simulink model "LS_5_Replication"  (R2022a)
settings: Solver=ode45  StartTime=0.0  StopTime=SIM_DURATION  RelTol=1e-3
PreLoadFcn:
  | SAMPLE_TIME = 0.01;
  | X1_0               = 3;
  | X2_0               = -1;
undefined symbols (not defined in the file): ACI_actor_proj_eps, ACI_alpha, ACI_beta1, ACI_eta_a1, ACI_eta_a2, ACI_eta_c, ACI_gamma, ACI_Gamma_0, ACI_Gamma_vf, ACI_Gamma_wf, ACI_k, ACI_mu, ACI_Q, ACI_R, ACI_Wa_max_proj, DiscIntNeverNeededParam, W_Actor_0, W_Critic_0, X_0, X_dilde_0
settings Model: Creator=Z0150218  LastModifiedBy=Z0150218

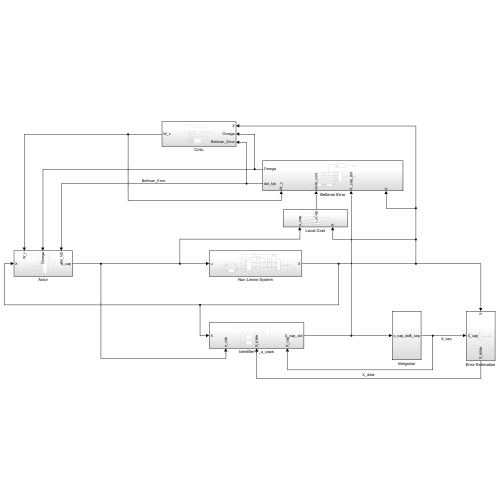
[thumbnail: Simulink's stored preview of the top-level diagram]
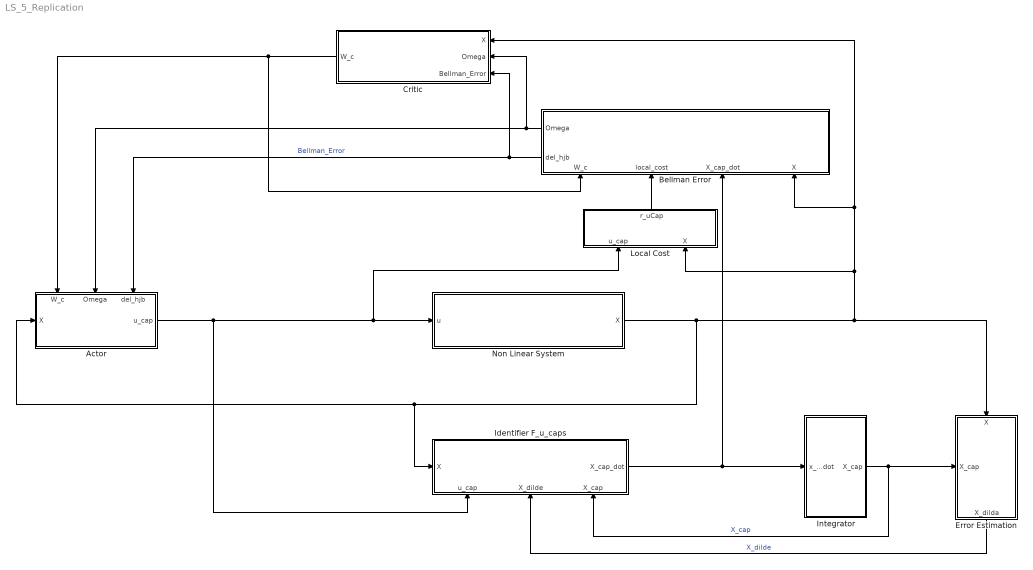
== system LS_5_Replication ==
  Actor : Subsystem
      settings: PortSchema="{\"entries\":[{\"content\":{\"sides\":[{\"content\":{\"connectorIds\":[\"In1\"]},\"type\":\"ConnectorPlacement.EquallySpacedRectSide\",\"uuid\":\"36bb19c7-ed28-4f81-a2b0-56b05d277fb3\"},{\"content\":{\"connectorIds\":[\"Out1\"],\"side\":\"RIGHT\"},\"type\":\"ConnectorPlacement.EquallySpacedRectSide\",\"uuid\":\"62e3b38d-27a4-411c-9c0c-4947886674bc\"},{\"content\":{\"connectorIds\":[\"In2\",\"In3\",\"In4\"],\"side\":\"TOP\"},\"type\":\"ConnectorPlacement.EquallySpacedRectSide\",\"uuid\":\"4750692c-c3eb-4933-9307-f150356a2a2d\"}]},\"type\":\"ConnectorPlacement.EquallySpacedConnector\",\"uuid\":\"9672208b-6d36-4217-80fb-cae3d46f9331\"}],\"packageUris\":[\"http://schema.mathworks.com/mf0/Connector/R2020b\"],\"version\":\"1.0\"}"
  Bellman Error : Subsystem
      settings: PortSchema="{\"entries\":[{\"content\":{\"sides\":[{\"content\":{\"connectorIds\":[]},\"type\":\"ConnectorPlacement.EquallySpacedRectSide\",\"uuid\":\"36bb19c7-ed28-4f81-a2b0-56b05d277fb3\"},{\"content\":{\"connectorIds\":[\"Out1\",\"Out2\"],\"side\":\"RIGHT\"},\"type\":\"ConnectorPlacement.EquallySpacedRectSide\",\"uuid\":\"62e3b38d-27a4-411c-9c0c-4947886674bc\"},{\"content\":{\"connectorIds\":[],\"side\":\"TOP\"},\"type\":\"ConnectorPlacement.EquallySpacedRectSide\",\"uuid\":\"4750692c-c3eb-4933-9307-f150356a2a2d\"},{\"content\":{\"connectorIds\":[\"In1\",\"In2\",\"In3\",\"In4\"],\"side\":\"BOTTOM\"},\"type\":\"ConnectorPlacement.EquallySpacedRectSide\",\"uuid\":\"b0657caa-1455-4a9e-81b4-6cca98e3a9da\"}]},\"type\":\"ConnectorPlacement.EquallySpacedConnector\",\"uuid\":\"9672208b-6d36-4217-80fb-cae3d46f9331\"}],\"packageUris\":[\"http://schema.mathworks.com/mf0/Connector/R2020b\"],\"version\":\"1.0\"}"
  Critic : Subsystem
  Error Estimation : Subsystem
      settings: PortSchema="{\"entries\":[{\"content\":{\"sides\":[{\"content\":{\"connectorIds\":[\"In1\"]},\"type\":\"ConnectorPlacement.EquallySpacedRectSide\",\"uuid\":\"e6cf2d84-7a10-4a43-bedd-b04786a9576e\"},{\"content\":{\"connectorIds\":[],\"side\":\"RIGHT\"},\"type\":\"ConnectorPlacement.EquallySpacedRectSide\",\"uuid\":\"10774151-562d-4d84-8145-e832c7227519\"},{\"content\":{\"connectorIds\":[\"In2\"],\"side\":\"TOP\"},\"type\":\"ConnectorPlacement.EquallySpacedRectSide\",\"uuid\":\"9da06394-e71b-407b-8c05-fa01b9a02c64\"},{\"content\":{\"connectorIds\":[\"Out1\"],\"side\":\"BOTTOM\"},\"type\":\"ConnectorPlacement.EquallySpacedRectSide\",\"uuid\":\"810c4029-0c70-4755-acf7-2aa0685db048\"}]},\"type\":\"ConnectorPlacement.EquallySpacedConnector\",\"uuid\":\"62376291-d5b3-4405-a096-61004334c23a\"}],\"packageUris\":[\"http://schema.mathworks.com/mf0/Connector/R2020b\"],\"version\":\"1.0\"}"
  Identifier F_u_caps : Subsystem
      settings: PortSchema="{\"entries\":[{\"content\":{\"sides\":[{\"content\":{\"connectorIds\":[\"In1\"]},\"type\":\"ConnectorPlacement.EquallySpacedRectSide\",\"uuid\":\"36bb19c7-ed28-4f81-a2b0-56b05d277fb3\"},{\"content\":{\"connectorIds\":[\"Out1\"],\"side\":\"RIGHT\"},\"type\":\"ConnectorPlacement.EquallySpacedRectSide\",\"uuid\":\"62e3b38d-27a4-411c-9c0c-4947886674bc\"},{\"content\":{\"connectorIds\":[],\"side\":\"TOP\"},\"type\":\"ConnectorPlacement.EquallySpacedRectSide\",\"uuid\":\"4750692c-c3eb-4933-9307-f150356a2a2d\"},{\"content\":{\"connectorIds\":[\"In2\",\"In3\",\"In4\"],\"side\":\"BOTTOM\"},\"type\":\"ConnectorPlacement.EquallySpacedRectSide\",\"uuid\":\"846bc86a-ab95-449a-8b91-40ba4137f590\"}]},\"type\":\"ConnectorPlacement.EquallySpacedConnector\",\"uuid\":\"9672208b-6d36-4217-80fb-cae3d46f9331\"}],\"packageUris\":[\"http://schema.mathworks.com/mf0/Connector/R2020b\"],\"version\":\"1.0\"}"
  Integrator : Subsystem
  Local Cost : Subsystem
      settings: PortSchema="{\"entries\":[{\"content\":{\"sides\":[{\"content\":{\"connectorIds\":[]},\"type\":\"ConnectorPlacement.EquallySpacedRectSide\",\"uuid\":\"36bb19c7-ed28-4f81-a2b0-56b05d277fb3\"},{\"content\":{\"connectorIds\":[],\"side\":\"RIGHT\"},\"type\":\"ConnectorPlacement.EquallySpacedRectSide\",\"uuid\":\"62e3b38d-27a4-411c-9c0c-4947886674bc\"},{\"content\":{\"connectorIds\":[\"Out1\"],\"side\":\"TOP\"},\"type\":\"ConnectorPlacement.EquallySpacedRectSide\",\"uuid\":\"4750692c-c3eb-4933-9307-f150356a2a2d\"},{\"content\":{\"connectorIds\":[\"In1\",\"In2\"],\"side\":\"BOTTOM\"},\"type\":\"ConnectorPlacement.EquallySpacedRectSide\",\"uuid\":\"45987bb4-5db5-4673-a5e8-75a3f7947a65\"}]},\"type\":\"ConnectorPlacement.EquallySpacedConnector\",\"uuid\":\"9672208b-6d36-4217-80fb-cae3d46f9331\"}],\"packageUris\":[\"http://schema.mathworks.com/mf0/Connector/R2020b\"],\"version\":\"1.0\"}"
  Non Linear System : Subsystem
  wires:
  Actor/1(u_cap) -> Non Linear System/1(u), Local Cost/1(u_cap), Identifier F_u_caps/2(u_cap)
  Identifier F_u_caps/1(X_cap_dot) -> Integrator/1(x_cap_dot), Bellman Error/2(X_cap_dot)
  Integrator/1(X_cap) -> Identifier F_u_caps/4(X_cap), Error Estimation/1(X_cap)  "X_cap"
  Non Linear System/1(X) -> Identifier F_u_caps/1(X), Actor/1(X), Bellman Error/1(X), Critic/1(X), Local Cost/2(X), Error Estimation/2(X)
  Critic/1(W_c) -> Actor/2(W_c), Bellman Error/4(W_c)
  Local Cost/1(r_uCap) -> Bellman Error/3(local_cost)
  Error Estimation/1(X_dilda) -> Identifier F_u_caps/3(X_dilde)  "X_dilde"
  Bellman Error/2(del_hjb) -> Critic/3(Bellman_Error), Actor/4(del_hjb)  "Bellman_Error"
  Bellman Error/1(Omega) -> Actor/3(Omega), Critic/2(Omega)

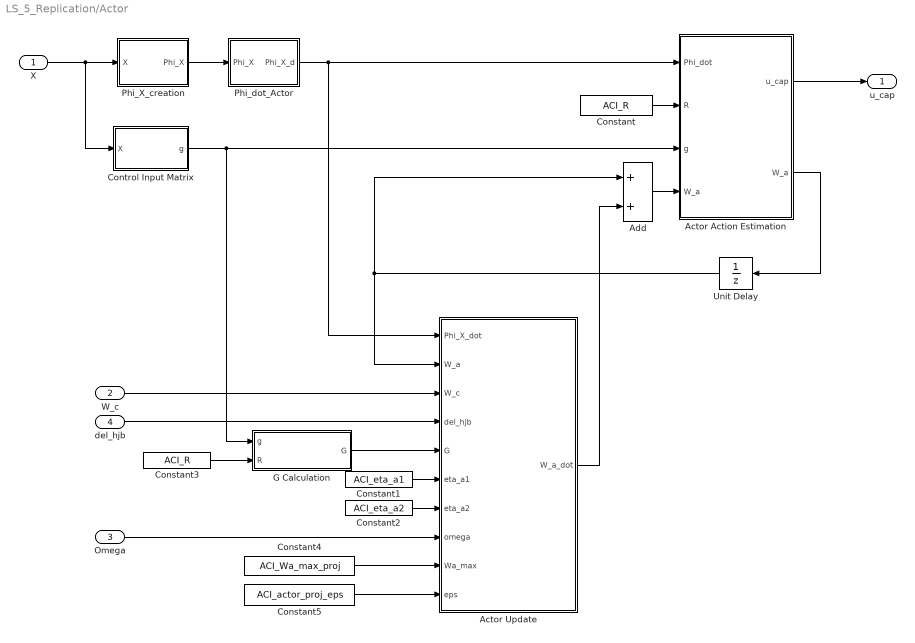
== system LS_5_Replication/Actor ==
  X : Inport
  W_c : Inport  Port=2
  Omega : Inport  Port=3
  del_hjb : Inport  Port=4
  Actor Action Estimation : MATLAB Function  TreatAsAtomicUnit=on
  Actor Update : MATLAB Function  TreatAsAtomicUnit=on
  Add : Sum
  Constant : Constant  Value=ACI_R
  Constant1 : Constant  Value=ACI_eta_a1
  Constant2 : Constant  Value=ACI_eta_a2
  Constant3 : Constant  Value=ACI_R
  Constant4 : Constant  Value=ACI_Wa_max_proj
  Constant5 : Constant  Value=ACI_actor_proj_eps
  Control Input Matrix : MATLAB Function  TreatAsAtomicUnit=on
  G Calculation : MATLAB Function  TreatAsAtomicUnit=on
  Phi_X_creation : MATLAB Function  TreatAsAtomicUnit=on
  Phi_dot_Actor : Subsystem
  Unit Delay : UnitDelay  InitialCondition=W_Actor_0  SampleTime=SAMPLE_TIME  HasFrameUpgradeWarning=on
  u_cap : Outport
  wires:
  Actor Action Estimation/2(W_a) -> Unit Delay/1
  Constant/1 -> Actor Action Estimation/2(R)
  Control Input Matrix/1(g) -> G Calculation/1(g), Actor Action Estimation/3(g)
  del_hjb/1 -> Actor Update/4(del_hjb)
  W_c/1 -> Actor Update/3(W_c)
  Unit Delay/1 -> Add/1, Actor Update/2(W_a)
  Actor Update/1(W_a_dot) -> Add/2
  Add/1 -> Actor Action Estimation/4("W_a ")
  X/1 -> Control Input Matrix/1(X), Phi_X_creation/1(X)
  Phi_X_creation/1(Phi_X) -> Phi_dot_Actor/1(Phi_X)
  Constant1/1 -> Actor Update/6(eta_a1)
  Constant2/1 -> Actor Update/7(eta_a2)
  Omega/1 -> Actor Update/8(omega)
  G Calculation/1(G) -> Actor Update/5(G)
  Constant3/1 -> G Calculation/2(R)
  Phi_dot_Actor/1(Phi_X_d) -> Actor Update/1(Phi_X_dot), Actor Action Estimation/1(Phi_dot)
  Actor Action Estimation/1(u_cap) -> u_cap/1
  Constant4/1 -> Actor Update/9(Wa_max)
  Constant5/1 -> Actor Update/10(eps)

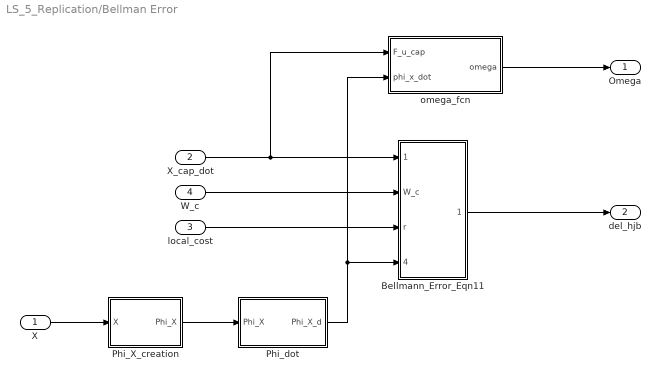
== system LS_5_Replication/Bellman Error ==
  X : Inport
  X_cap_dot : Inport  Port=2
  local_cost : Inport  Port=3
  W_c : Inport  Port=4
  Bellmann_Error_Eqn11 : MATLAB Function  TreatAsAtomicUnit=on
  Phi_X_creation : MATLAB Function  TreatAsAtomicUnit=on
  Phi_dot : Subsystem
  omega_fcn : MATLAB Function  TreatAsAtomicUnit=on
  Omega : Outport
  del_hjb : Outport  Port=2
  wires:
  X/1 -> Phi_X_creation/1(X)
  Phi_X_creation/1(Phi_X) -> Phi_dot/1(Phi_X)
  local_cost/1 -> Bellmann_Error_Eqn11/3(r)
  W_c/1 -> Bellmann_Error_Eqn11/2(W_c)
  X_cap_dot/1 -> Bellmann_Error_Eqn11/1(F_u_cap), omega_fcn/1(F_u_cap)
  Bellmann_Error_Eqn11/1(del_hjb) -> del_hjb/1
  Phi_dot/1(Phi_X_d) -> Bellmann_Error_Eqn11/4(phi_x_d), omega_fcn/2(phi_x_dot)
  omega_fcn/1(omega) -> Omega/1

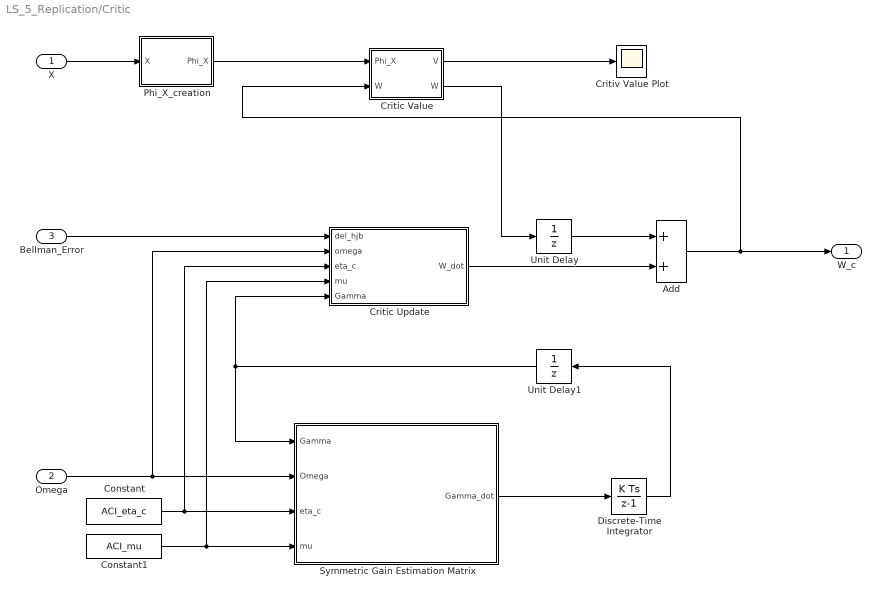
== system LS_5_Replication/Critic ==
  X : Inport
  Omega : Inport  Port=2
  Bellman_Error : Inport  Port=3
  Add : Sum
  Constant : Constant  Value=ACI_eta_c
  Constant1 : Constant  Value=ACI_mu
  Critic Update : MATLAB Function  TreatAsAtomicUnit=on
  Critic Value : MATLAB Function  TreatAsAtomicUnit=on
  Critiv Value Plot : Scope
  Discrete-Time Integrator : DiscreteIntegrator  InitialCondition=ACI_Gamma_0  SampleTime=-1  ICPrevOutput=DiscIntNeverNeededParam  ICPrevScaledInput=DiscIntNeverNeededParam
  Phi_X_creation : MATLAB Function  TreatAsAtomicUnit=on
  Symmetric Gain Estimation Matrix : MATLAB Function  TreatAsAtomicUnit=on
  Unit Delay : UnitDelay  InitialCondition=W_Critic_0  SampleTime=SAMPLE_TIME  HasFrameUpgradeWarning=on
  Unit Delay1 : UnitDelay  SampleTime=-1  HasFrameUpgradeWarning=on
  W_c : Outport
  wires:
  Critic Value/1(V) -> Critiv Value Plot/1
  Add/1 -> Critic Value/2("W "), W_c/1
  X/1 -> Phi_X_creation/1(X)
  Critic Value/2(W) -> Unit Delay/1
  Critic Update/1(W_dot) -> Add/2
  Bellman_Error/1 -> Critic Update/1(del_hjb)
  Unit Delay/1 -> Add/1
  Phi_X_creation/1(Phi_X) -> Critic Value/1(Phi_X)
  Symmetric Gain Estimation Matrix/1(Gamma_dot) -> Discrete-Time Integrator/1
  Discrete-Time Integrator/1 -> Unit Delay1/1
  Omega/1 -> Critic Update/2(omega), Symmetric Gain Estimation Matrix/2(Omega)
  Constant/1 -> Critic Update/3(eta_c), Symmetric Gain Estimation Matrix/3(eta_c)
  Constant1/1 -> Critic Update/4(mu), Symmetric Gain Estimation Matrix/4(mu)
  Unit Delay1/1 -> Critic Update/5(Gamma), Symmetric Gain Estimation Matrix/1(Gamma)

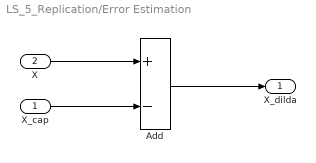
== system LS_5_Replication/Error Estimation ==
  X_cap : Inport
  X : Inport  Port=2
  Add : Sum  Inputs=+-
  X_dilda : Outport
  wires:
  Add/1 -> X_dilda/1
  X/1 -> Add/1
  X_cap/1 -> Add/2

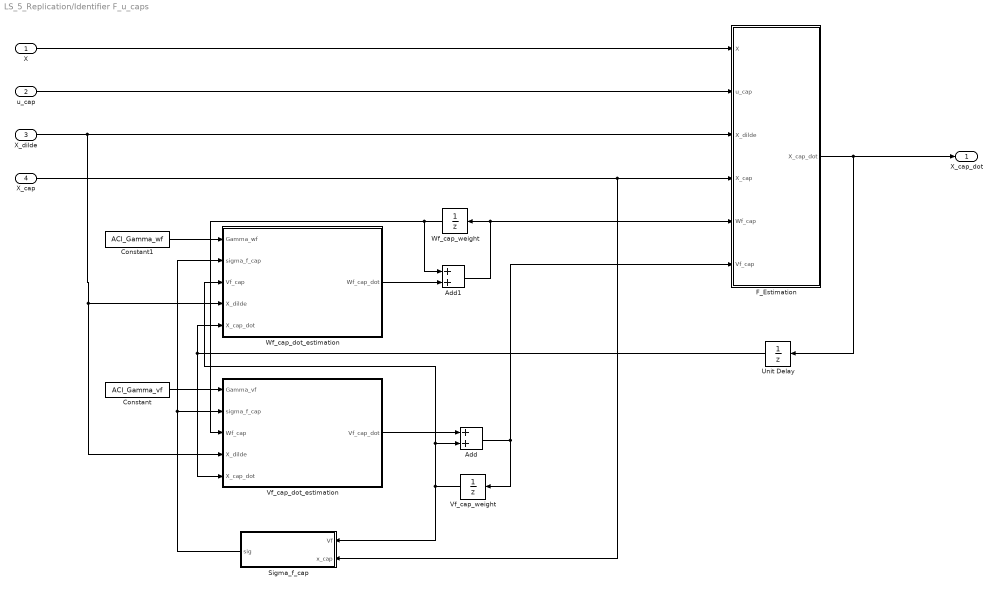
== system LS_5_Replication/Identifier F_u_caps ==
  X : Inport
  u_cap : Inport  Port=2
  X_dilde : Inport  Port=3
  X_cap : Inport  Port=4
  Add : Sum
  Add1 : Sum
  Constant : Constant  Value=ACI_Gamma_vf
  Constant1 : Constant  Value=ACI_Gamma_wf
  F_Estimation : Subsystem
  Sigma_f_cap : MATLAB Function  TreatAsAtomicUnit=on
  Unit Delay : UnitDelay  SampleTime=-1  HasFrameUpgradeWarning=on
  Vf_cap_dot_estimation : MATLAB Function  TreatAsAtomicUnit=on
  Vf_cap_weight : UnitDelay  SampleTime=-1  HasFrameUpgradeWarning=on
  Wf_cap_dot_estimation : MATLAB Function  TreatAsAtomicUnit=on
  Wf_cap_weight : UnitDelay  SampleTime=-1  HasFrameUpgradeWarning=on
  X_cap_dot : Outport
  wires:
  u_cap/1 -> F_Estimation/2(u_cap)
  X_dilde/1 -> Vf_cap_dot_estimation/4(X_dilde), Wf_cap_dot_estimation/4(X_dilde), F_Estimation/3(X_dilde)
  X_cap/1 -> Sigma_f_cap/2(x_cap), F_Estimation/4(X_cap)
  Wf_cap_dot_estimation/1(Wf_cap_dot) -> Add1/2
  Constant1/1 -> Wf_cap_dot_estimation/1(Gamma_wf)
  Vf_cap_dot_estimation/1(Vf_cap_dot) -> Add/1
  Constant/1 -> Vf_cap_dot_estimation/1(Gamma_vf)
  Add/1 -> F_Estimation/6(Vf_cap), Vf_cap_weight/1
  Add1/1 -> Wf_cap_weight/1, F_Estimation/5(Wf_cap)
  Vf_cap_weight/1 -> Wf_cap_dot_estimation/3(Vf_cap), Add/2, Sigma_f_cap/1(Vf)
  Wf_cap_weight/1 -> Add1/1, Vf_cap_dot_estimation/3(Wf_cap)
  X/1 -> F_Estimation/1(X)
  Sigma_f_cap/1(sig) -> Vf_cap_dot_estimation/2(sigma_f_cap), Wf_cap_dot_estimation/2(sigma_f_cap)
  F_Estimation/1(X_cap_dot) -> X_cap_dot/1, Unit Delay/1
  Unit Delay/1 -> Vf_cap_dot_estimation/5(X_cap_dot), Wf_cap_dot_estimation/5(X_cap_dot)

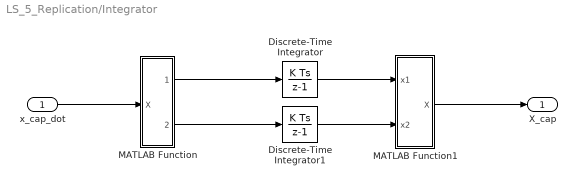
== system LS_5_Replication/Integrator ==
  x_cap_dot : Inport
  Discrete-Time Integrator : DiscreteIntegrator  SampleTime=SAMPLE_TIME  ICPrevOutput=DiscIntNeverNeededParam  ICPrevScaledInput=DiscIntNeverNeededParam
  Discrete-Time Integrator1 : DiscreteIntegrator  SampleTime=SAMPLE_TIME  ICPrevOutput=DiscIntNeverNeededParam  ICPrevScaledInput=DiscIntNeverNeededParam
  MATLAB Function : MATLAB Function  TreatAsAtomicUnit=on
  MATLAB Function1 : MATLAB Function  TreatAsAtomicUnit=on
  X_cap : Outport
  wires:
  x_cap_dot/1 -> MATLAB Function/1(X)
  MATLAB Function/1(x1) -> Discrete-Time Integrator/1
  MATLAB Function/2(x2) -> Discrete-Time Integrator1/1
  Discrete-Time Integrator/1 -> MATLAB Function1/1(x1)
  Discrete-Time Integrator1/1 -> MATLAB Function1/2(x2)
  MATLAB Function1/1(X) -> X_cap/1

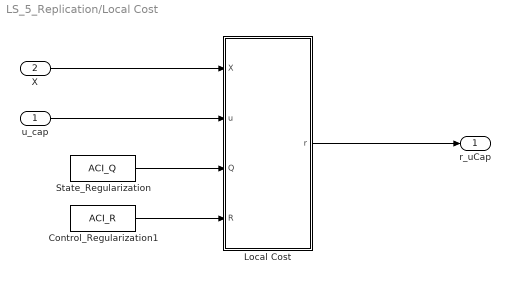
== system LS_5_Replication/Local Cost ==
  u_cap : Inport
  X : Inport  Port=2
  Control_Regularization1 : Constant  Value=ACI_R
  Local Cost : MATLAB Function  TreatAsAtomicUnit=on
  State_Regularization : Constant  Value=ACI_Q
  r_uCap : Outport
  wires:
  u_cap/1 -> Local Cost/2(u)
  X/1 -> Local Cost/1(X)
  State_Regularization/1 -> Local Cost/3(Q)
  Control_Regularization1/1 -> Local Cost/4(R)
  Local Cost/1(r) -> r_uCap/1

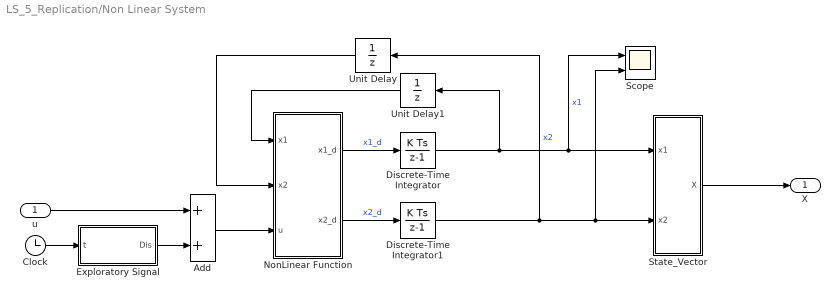
== system LS_5_Replication/Non Linear System ==
  u : Inport
  Add : Sum
  Clock : Clock
  Discrete-Time Integrator : DiscreteIntegrator  InitialCondition=X_0(1)  SampleTime=SAMPLE_TIME  ICPrevOutput=DiscIntNeverNeededParam  ICPrevScaledInput=DiscIntNeverNeededParam
  Discrete-Time Integrator1 : DiscreteIntegrator  InitialCondition=X_0(2)  SampleTime=SAMPLE_TIME  ICPrevOutput=DiscIntNeverNeededParam  ICPrevScaledInput=DiscIntNeverNeededParam
  Exploratory Signal : MATLAB Function  TreatAsAtomicUnit=on
  NonLinear Function : MATLAB Function  TreatAsAtomicUnit=on
  Scope : Scope  NumInputPorts=2
  State_Vector : MATLAB Function  TreatAsAtomicUnit=on
  Unit Delay : UnitDelay  SampleTime=-1  HasFrameUpgradeWarning=on
  Unit Delay1 : UnitDelay  SampleTime=-1  HasFrameUpgradeWarning=on
  X : Outport
  wires:
  Discrete-Time Integrator1/1 -> Unit Delay/1, Scope/2, State_Vector/2(x2)  "x2"
  NonLinear Function/2(x2_d) -> Discrete-Time Integrator1/1  "x2_d"
  NonLinear Function/1(x1_d) -> Discrete-Time Integrator/1  "x1_d"
  Discrete-Time Integrator/1 -> State_Vector/1(x1), Scope/1, Unit Delay1/1  "x1"
  State_Vector/1(X) -> X/1
  u/1 -> Add/1
  Unit Delay1/1 -> NonLinear Function/1(x1)
  Unit Delay/1 -> NonLinear Function/2(x2)
  Clock/1 -> Exploratory Signal/1(t)
  Exploratory Signal/1(Dis) -> Add/2
  Add/1 -> NonLinear Function/3(u)

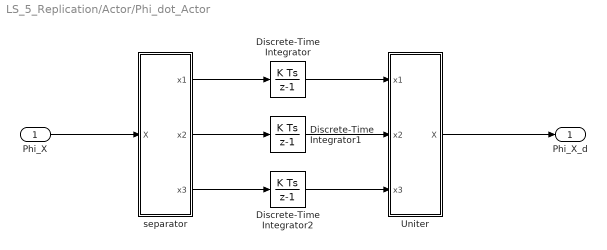
== system LS_5_Replication/Actor/Phi_dot_Actor ==
  Phi_X : Inport
  Discrete-Time Integrator : DiscreteIntegrator  SampleTime=-1  ICPrevOutput=DiscIntNeverNeededParam  ICPrevScaledInput=DiscIntNeverNeededParam
  Discrete-Time Integrator1 : DiscreteIntegrator  SampleTime=-1  ICPrevOutput=DiscIntNeverNeededParam  ICPrevScaledInput=DiscIntNeverNeededParam
  Discrete-Time Integrator2 : DiscreteIntegrator  SampleTime=-1  ICPrevOutput=DiscIntNeverNeededParam  ICPrevScaledInput=DiscIntNeverNeededParam
  Uniter : MATLAB Function  TreatAsAtomicUnit=on
  separator : MATLAB Function  TreatAsAtomicUnit=on
  Phi_X_d : Outport
  wires:
  Phi_X/1 -> separator/1(X)
  separator/1(x1) -> Discrete-Time Integrator/1
  separator/3(x3) -> Discrete-Time Integrator2/1
  separator/2(x2) -> Discrete-Time Integrator1/1
  Discrete-Time Integrator/1 -> Uniter/1(x1)
  Discrete-Time Integrator1/1 -> Uniter/2(x2)
  Discrete-Time Integrator2/1 -> Uniter/3(x3)
  Uniter/1(X) -> Phi_X_d/1

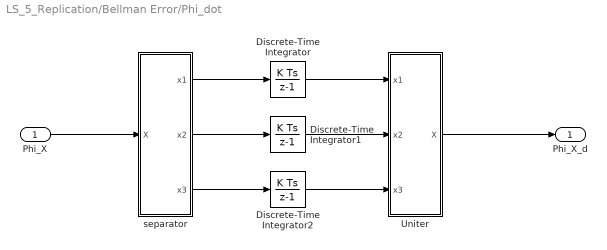
== system LS_5_Replication/Bellman Error/Phi_dot ==
  Phi_X : Inport
  Discrete-Time Integrator : DiscreteIntegrator  SampleTime=-1  ICPrevOutput=DiscIntNeverNeededParam  ICPrevScaledInput=DiscIntNeverNeededParam
  Discrete-Time Integrator1 : DiscreteIntegrator  SampleTime=-1  ICPrevOutput=DiscIntNeverNeededParam  ICPrevScaledInput=DiscIntNeverNeededParam
  Discrete-Time Integrator2 : DiscreteIntegrator  SampleTime=-1  ICPrevOutput=DiscIntNeverNeededParam  ICPrevScaledInput=DiscIntNeverNeededParam
  Uniter : MATLAB Function  TreatAsAtomicUnit=on
  separator : MATLAB Function  TreatAsAtomicUnit=on
  Phi_X_d : Outport
  wires:
  Phi_X/1 -> separator/1(X)
  separator/1(x1) -> Discrete-Time Integrator/1
  separator/3(x3) -> Discrete-Time Integrator2/1
  separator/2(x2) -> Discrete-Time Integrator1/1
  Discrete-Time Integrator/1 -> Uniter/1(x1)
  Discrete-Time Integrator1/1 -> Uniter/2(x2)
  Discrete-Time Integrator2/1 -> Uniter/3(x3)
  Uniter/1(X) -> Phi_X_d/1

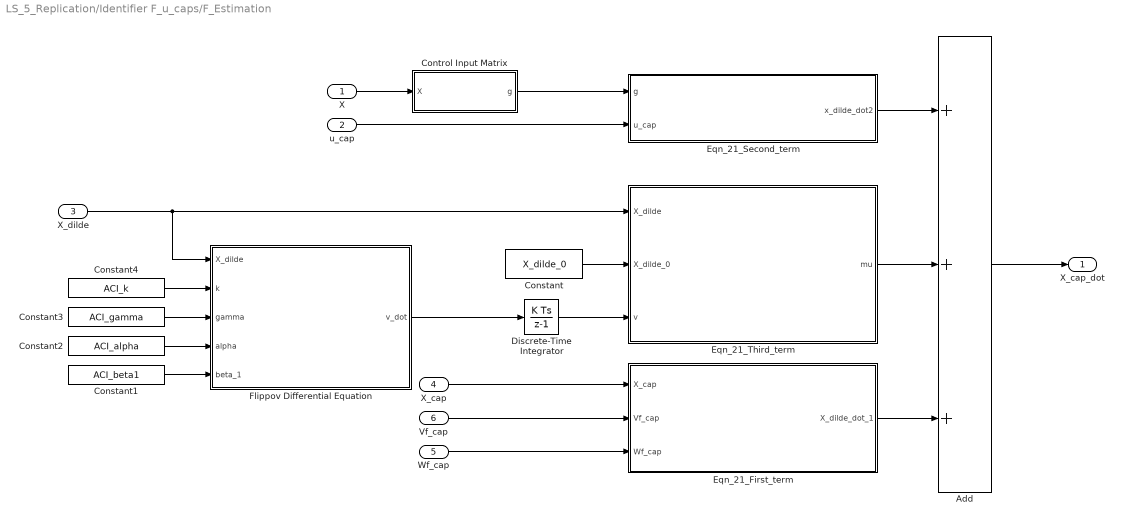
== system LS_5_Replication/Identifier F_u_caps/F_Estimation ==
  X : Inport
  u_cap : Inport  Port=2
  X_dilde : Inport  Port=3
  X_cap : Inport  Port=4
  Wf_cap : Inport  Port=5
  Vf_cap : Inport  Port=6
  Add : Sum  Inputs=+++
  Constant : Constant  Value=X_dilde_0
  Constant1 : Constant  Value=ACI_beta1
  Constant2 : Constant  Value=ACI_alpha
  Constant3 : Constant  Value=ACI_gamma
  Constant4 : Constant  Value=ACI_k
  Control Input Matrix : MATLAB Function  TreatAsAtomicUnit=on
  Discrete-Time Integrator : DiscreteIntegrator  SampleTime=SAMPLE_TIME  ICPrevOutput=DiscIntNeverNeededParam  ICPrevScaledInput=DiscIntNeverNeededParam
  Eqn_21_First_term : MATLAB Function  TreatAsAtomicUnit=on
  Eqn_21_Second_term : MATLAB Function  TreatAsAtomicUnit=on
  Eqn_21_Third_term : MATLAB Function  TreatAsAtomicUnit=on
  Flippov Differential Equation : MATLAB Function  TreatAsAtomicUnit=on
  X_cap_dot : Outport
  wires:
  Vf_cap/1 -> Eqn_21_First_term/2(Vf_cap)
  X_dilde/1 -> Flippov Differential Equation/1(X_dilde), Eqn_21_Third_term/1(X_dilde)
  Discrete-Time Integrator/1 -> Eqn_21_Third_term/3(v)
  Eqn_21_Second_term/1(x_dilde_dot2) -> Add/1
  X_cap/1 -> Eqn_21_First_term/1(X_cap)
  Constant/1 -> Eqn_21_Third_term/2(X_dilde_0)
  Eqn_21_First_term/1(X_dilde_dot_1) -> Add/3
  Flippov Differential Equation/1(v_dot) -> Discrete-Time Integrator/1
  Eqn_21_Third_term/1(mu) -> Add/2
  Add/1 -> X_cap_dot/1
  Wf_cap/1 -> Eqn_21_First_term/3(Wf_cap)
  u_cap/1 -> Eqn_21_Second_term/2(u_cap)
  X/1 -> Control Input Matrix/1(X)
  Control Input Matrix/1(g) -> Eqn_21_Second_term/1(g)
  Constant1/1 -> Flippov Differential Equation/5(beta_1)
  Constant2/1 -> Flippov Differential Equation/4(alpha)
  Constant3/1 -> Flippov Differential Equation/3(gamma)
  Constant4/1 -> Flippov Differential Equation/2(k)

== matlab function LS_5_Replication/Identifier F_u_caps/F_Estimation/Flippov Differential Equation ==
  data: X_dilde input; v_dot output; k input; gamma input; alpha input; beta_1 input
function v_dot = Flippov_GS(X_dilde, k, gamma, alpha, beta_1)

v_dot_1                = ((k*alpha) + gamma) * X_dilde;
v_dot_2                = beta_1 * sign(X_dilde);
v_dot                  = v_dot_1 + v_dot_2;

== matlab function LS_5_Replication/Identifier F_u_caps/F_Estimation/Eqn_21_First_term ==
  data: X_cap input; X_dilde_dot_1 output; Vf_cap input; Wf_cap input
function X_dilde_dot_1  = DNN(X_cap, Vf_cap, Wf_cap)

term1            = Vf_cap'*X_cap;
sigma_f_cap      = fcn_ACI_DNN_Activation(term1);
X_dilde_dot_1    = Wf_cap'*sigma_f_cap;
end

== matlab function LS_5_Replication/Identifier F_u_caps/Wf_cap_dot_estimation ==
  data: Gamma_wf input; Wf_cap_dot output; sigma_f_cap input; Vf_cap input; X_dilde input; X_cap_dot input
function Wf_cap_dot = Wf_cap_d_Est(Gamma_wf, sigma_f_cap,Vf_cap,X_dilde,X_cap_dot)


Proj              = 1;
Wf_cap_dot_t      = Proj*Gamma_wf*sigma_f_cap'*Vf_cap'*X_cap_dot*X_dilde';
Wf_cap_dot        = Wf_cap_dot_t;
end

== matlab function LS_5_Replication/Identifier F_u_caps/Vf_cap_dot_estimation ==
  data: Gamma_vf input; Vf_cap_dot output; sigma_f_cap input; Wf_cap input; X_dilde input; X_cap_dot input
function Vf_cap_dot = Vf_cap_d_Est(Gamma_vf, sigma_f_cap,Wf_cap,X_dilde,X_cap_dot)


Proj              = 1;
Vf_cap_dot        = Proj*Gamma_vf*X_cap_dot*X_dilde'*Wf_cap'*sigma_f_cap';

end

== matlab function LS_5_Replication/Local Cost/Local Cost ==
  data: X input; u input; r output; Q input; R input
function r = Local_Cost(X,u,Q,R)

elem1     = u'*R*u;
elem2     = X'*Q*X;
r         = elem1 + elem2;
end

== matlab function LS_5_Replication/Bellman Error/Bellmann_Error_Eqn11 ==
  data: F_u_cap input; W_c input; del_hjb output; r input; phi_x_d input
function del_hjb = hjb(F_u_cap,W_c,r,phi_x_d)

omega   = phi_x_d * F_u_cap; 
del_hjb = (W_c'*omega) + r;
end

== matlab function LS_5_Replication/Critic/Critic Value ==
  data: Phi_X input; W input; V output; W output
function [V,W] = Critic(Phi_X,W)


V     = W'*Phi_X;  % Equation 10
end

== matlab function LS_5_Replication/Integrator/MATLAB Function ==
  data: X input; x1 output; x2 output
function [x1,x2] = fcn(X)

x1 = X(1);
x2 = X(2);
end

== matlab function LS_5_Replication/Integrator/MATLAB Function1 ==
  data: x1 input; X output; x2 input
function X = fcn(x1,x2)

X = [x1; x2];

== matlab function LS_5_Replication/Bellman Error/Phi_X_creation ==
  data: X input; Phi_X output
function Phi_X = fcn_ACI_Phi(X)
px1   = X(1)^2;
px2   = X(1)*X(2);
px3   = X(2)^2;
Phi_X = [px1; px2; px3];

end

== matlab function LS_5_Replication/Bellman Error/Phi_dot/separator ==
  data: X input; x1 output; x2 output; x3 output
function [x1,x2,x3] = fcn(X)

x1 = X(1);
x2 = X(2);
x3 = X(3);
end

== matlab function LS_5_Replication/Bellman Error/Phi_dot/Uniter ==
  data: x1 input; X output; x2 input; x3 input
function X  = fcn(x1,x2,x3)

X = [x1 x1; x2 x2; x3 x3];
end

== matlab function LS_5_Replication/Non Linear System/State_Vector ==
  data: x1 input; X output; x2 input
function X = fcn(x1,x2)

X = [x1; x2];

end

== matlab function LS_5_Replication/Critic/Phi_X_creation ==
  data: X input; Phi_X output
function Phi_X = fcn_ACI_Phi(X)
px1   = X(1)^2;
px2   = X(1)*X(2);
px3   = X(2)^2;
Phi_X = [px1; px2; px3];

end

== matlab function LS_5_Replication/Actor/Phi_X_creation ==
  data: X input; Phi_X output
function Phi_X = fcn_ACI_Phi(X)
px1   = X(1)^2;
px2   = X(1)*X(2);
px3   = X(2)^2;
Phi_X = [px1; px2; px3];

end

== matlab function LS_5_Replication/Critic/Symmetric Gain Estimation Matrix ==
  data: Gamma input; Gamma_dot output; Omega input; eta_c input; mu input
function Gamma_dot = Gain_Matrix(Gamma,Omega,eta_c,mu)

num         = Omega*Omega';
den         = 1 + (mu*Omega'*Gamma*Omega);

temp        = num/den;

Gamma_dot   = -eta_c*Gamma*temp*Gamma;


end

== matlab function LS_5_Replication/Bellman Error/omega_fcn ==
  data: F_u_cap input; phi_x_dot input; omega output
function omega = fcn(F_u_cap, phi_x_dot)

omega = phi_x_dot*F_u_cap;
end

== matlab function LS_5_Replication/Actor/Phi_dot_Actor/Uniter ==
  data: x1 input; X output; x2 input; x3 input
function X  = fcn(x1,x2,x3)

X = [x1 x1; x2 x2; x3 x3];
end

== matlab function LS_5_Replication/Non Linear System/NonLinear Function ==
  data: x1 input; x2 input; u input; x1_d output; x2_d output
function [x1_d, x2_d] = Non_Linear(x1,x2,u)

x1_d = -x1 + x2;
x2_d = (-0.5*x1) - (0.5*x2*(1 - (cos(2*x1)+2)^2)) + (cos(2*x1)+2)*u;
end

== matlab function LS_5_Replication/Actor/Phi_dot_Actor/separator ==
  data: X input; x1 output; x2 output; x3 output
function [x1,x2,x3] = fcn(X)

x1 = X(1);
x2 = X(2);
x3 = X(3);
end

== matlab function LS_5_Replication/Actor/G Calculation ==
  data: g input; G output; R input
function G = G_symmetric(g,R)

term1 = R\g;
G     = term1*g';
end

== matlab function LS_5_Replication/Non Linear System/Exploratory Signal ==
  data: t input; Dis output
function Dis = PE(t)

if t <= 3
    tm1 = cos(t)*(sin(t)^2);
    tm2 = cos(0.1*t)*(sin(2*t)^2);
    tm3 = cos(0.5*t)*(sin(-1.2*t)^2);
    tm4 = sin(t)^5;
    Dis = tm1 + tm2 +tm3 + tm4;
else
    Dis = 0;
end

== matlab function LS_5_Replication/Identifier F_u_caps/Sigma_f_cap ==
  data: Vf input; sig output; x_cap input
function sig = Sigma_f_cap(Vf,x_cap)

sig = fcn_ACI_DNN_Activation(Vf'*x_cap);
end

== matlab function LS_5_Replication/Critic/Critic Update ==
  data: del_hjb input; omega input; eta_c input; mu input; W_dot output; Gamma input
function W_dot = Critic_Update(del_hjb, omega,eta_c,  mu, Gamma)

num     = -eta_c*Gamma*omega*del_hjb;
den     = 1 + mu*omega'*Gamma*omega;
W_dot   = num./den;
end

== matlab function LS_5_Replication/Actor/Actor Action Estimation ==
  data: Phi_dot input; R input; g input; u_cap output; W_a input; W_a output
function [u_cap, W_a] = Actor_Action(Phi_dot,R,g,W_a)

u_cap       = -0.5*g'*Phi_dot'*W_a\R;     % Equation 10 -s

== matlab function LS_5_Replication/Actor/Control Input Matrix ==
  data: X input; g output
function g = Control_Input(X)
x1  = 0;
x2  = cos(2*X(1)) + 2;

g   = [x1; x2];

== matlab function LS_5_Replication/Actor/Actor Update ==
  data: Phi_X_dot input; W_a input; W_a_dot output; W_c input; del_hjb input; G input; eta_a1 input; eta_a2 input; omega input; Wa_max input; eps input
function W_a_dot = Actor_Update(Phi_X_dot, W_a, W_c, del_hjb, G, eta_a1, eta_a2,omega, Wa_max, eps)


term1_den      = sqrt(1 + (omega'*omega));
term1_num      = -eta_a1*Phi_X_dot*G*Phi_X_dot'*(W_a - W_c)*del_hjb;
term1          = term1_num./term1_den;

term2          = -eta_a2*(W_a - W_c);                    

W_a_dot_uproj = term1 + term2;                              % Equation 39

W_a_dot        = W_a_dot_uproj; %fcn_ACI_proj(W_a, W_a_dot_uproj, Wa_max, eps);


end

== matlab function LS_5_Replication/Identifier F_u_caps/F_Estimation/Control Input Matrix ==
  data: X input; g output
function g = Control_Input(X)
x1     = 0;
x2     = cos(2*X(1)) + 2;
g     = [x1; x2];
end

== matlab function LS_5_Replication/Identifier F_u_caps/F_Estimation/Eqn_21_Second_term ==
  data: g input; x_dilde_dot2 output; u_cap input
function x_dilde_dot2 = gx_times_u(g,u_cap)

x_dilde_dot2 = g*u_cap;

== matlab function LS_5_Replication/Identifier F_u_caps/F_Estimation/Eqn_21_Third_term ==
  data: X_dilde input; mu output; X_dilde_0 input; v input
function mu = RISE_feedback(X_dilde,X_dilde_0, v)

k    = 1 ; % positive contant gains


mu = (k*X_dilde) + (k*X_dilde_0) + v; % Equation 22
